simulink model "VehCtrlMdel241025_2018b_amkspdlimit"  (R2019b)
settings: Solver=FixedStepDiscrete  StartTime=0.0  StopTime=30  FixedStep=0.0005  RelTol=1e-3  EnableMultiTasking=on
values from neighbouring files (symbols this model uses):
  Ldwf = 0.4    [VxSpdEstiPara.m]
  Ldwr = 0.5    [VxSpdEstiPara.m]
  thr1 = 0.5    [VxSpdEstiPara.m]
  thr2 = 0.5    [VxSpdEstiPara.m]
  thr3 = 0.5    [VxSpdEstiPara.m]
  thr4 = 0.5    [VxSpdEstiPara.m]
  TrqRquRate = 20    [VxSpdEstiPara.m]
undefined symbols (not defined in the file or in its folder): Ax_OffSet, Ay_OffSet, Caf, Car, DiscIntNeverNeededParam, dwf, dwr, h, i1, i2, I_AN06_5V, I_AN07_5V, I_AN08_5V, I_AN09_5V, I_AN10_5V, I_SW01_L, I_SW02_L, I_SW03_L, I_SW05_L, I_SW07_L, Iz, Kc, Ki, Kp, lf, lr, m, O_SW01_LS0A4, O_SW02_LS0A4, O_SW04_LS0A4, O_SW05_LS0A4, O_SW06_LS0A4, O_SW07_LS0A4, O_SW08_LS0A4, O_SW09_LS0A4, O_SW12_HS1A, O_SW13_HS1A, O_SW14_HS1A, O_SW15_HS1A, Offset_Angle, PWM3, Qa, Ra, RearRatio, Rt, thr5, YawRate_OffSet
libraries: simulink x159, ec5744lib x142, canmsglib x18, MyDesignedModel x1
(part 2 of 6)

== system VehCtrlMdel241025_2018b_amkspdlimit/Input/key ==
  note: 1:cutoff
  function : TriggerPort  TriggerType=function-call  VariantControl=(inherit)
  Acc4 : ec5744lib/RapidECU_U3/01BasicInput/AnalogInput  channel=56:I_AN10_5V  sampletime=-1
      settings: SourceProductName=ECUCoder for MPC5744
  Bus Creator : BusCreator  Inputs=6
  Compare To Constant : simulink/Logic and Bit Operations/Compare To Constant  relop=<=  const=1500  OutDataTypeStr=boolean
  Constant1 : Constant  Value=single(0.11)
  Constant2 : Constant  Commented=on  Value=boolean(1)
  Constant3 : Constant  Value=single(0.11)
  Constant5 : Constant  Value=single(0.11)
  Logical Operator : Logic  Operator=NOT  AllPortsSameDT=off  OutDataTypeStr=boolean
  MeaModule : ec5744lib/RapidECU_U3/07Calibration/MeaModule  signal=TSAL_SW_IN
      settings: SourceProductName=ECUCoder for MPC5744
  MeaModule1 : ec5744lib/RapidECU_U3/07Calibration/MeaModule  signal=ignition
      settings: SourceProductName=ECUCoder for MPC5744
  MeaModule2 : ec5744lib/RapidECU_U3/07Calibration/MeaModule  signal=AMKSWITCH
      settings: SourceProductName=ECUCoder for MPC5744
  MeaModule3 : ec5744lib/RapidECU_U3/07Calibration/MeaModule  signal=HV_voltValid
      settings: SourceProductName=ECUCoder for MPC5744
  SwitchInput : ec5744lib/RapidECU_U3/01BasicInput/SwitchInput  channel=7:I_SW02_L  sampletime=-1
      settings: SourceProductName=ECUCoder for MPC5744
  SwitchInput1 : ec5744lib/RapidECU_U3/01BasicInput/SwitchInput  channel=8:I_SW03_L  sampletime=-1
      settings: SourceProductName=ECUCoder for MPC5744
  SwitchInput2 : ec5744lib/RapidECU_U3/01BasicInput/SwitchInput  channel=10:I_SW05_L  sampletime=-1
      settings: SourceProductName=ECUCoder for MPC5744
  SwitchInput3 : ec5744lib/RapidECU_U3/01BasicInput/SwitchInput  channel=6:I_SW01_L  sampletime=-1
      settings: SourceProductName=ECUCoder for MPC5744
  SwitchInput4 : ec5744lib/RapidECU_U3/01BasicInput/SwitchInput  channel=26:I_SW07_L  sampletime=-1
      settings: SourceProductName=ECUCoder for MPC5744
  Timer : Stateflow chart  TreatAsAtomicUnit=on
  Timer1 : Stateflow chart  TreatAsAtomicUnit=on
  Timer2 : Stateflow chart  TreatAsAtomicUnit=on
  key : Outport  VectorParamsAs1DForOutWhenUnconnected=off
  wires:
  SwitchInput/1 -> Logical Operator/1  "Drive_ready"
  Bus Creator/1 -> key/1
  Logical Operator/1 -> Timer/1(Trigger)  "ignition"
  Constant5/1 -> Timer/2(CountTime)
  Timer/1(Exit) -> MeaModule1/1  "ignition"
  MeaModule1/1 -> Bus Creator/1
  Constant1/1 -> Timer1/2(CountTime)
  Timer1/1(Exit) -> MeaModule2/1  "AMKSWITCH"
  MeaModule2/1 -> Bus Creator/2
  SwitchInput3/1 -> Bus Creator/3  "out2"
  SwitchInput1/1 -> Timer1/1(Trigger)
  Acc4/1 -> Compare To Constant/1  "HV_volt"
  MeaModule/1 -> Bus Creator/4  "TSAL_SW_IN"
  MeaModule3/1 -> Bus Creator/5  "HV_voltValid"
  Compare To Constant/1 -> MeaModule3/1
  SwitchInput4/1 -> Timer2/1(Trigger)
  Timer2/1(Exit) -> Bus Creator/6  "ModeSW"
  Constant3/1 -> Timer2/2(CountTime)
  SwitchInput2/1 -> MeaModule/1  "ignition"

== system VehCtrlMdel241025_2018b_amkspdlimit/Input_Processing/Function-Call Subsystem ==
  INPUT_BUS : Inport
  function : TriggerPort  TriggerType=function-call  VariantControl=Variant
  AccBrkPedal : Subsystem
  Bus Selector : BusSelector  OutputSignals=IMU,AccBrk_BUS,SWAS,ABS_BUS,AMKMCUtoVCU_BUS,AMKMCUtoVCU_BUS.FLAMKMCUtoVCU1,AMKMCUtoVCU_BUS.FRAMKMCUtoVCU1,EMRAXMCU_Receive.MCU_pwr
  Bus Creator : BusCreator  Inputs=6
  IMU : Subsystem
  SWAS : Subsystem
  Subsystem : Subsystem
  Subsystem1 : Subsystem
  Terminator : Terminator
  Terminator1 : Terminator
  Terminator2 : Terminator
  WhlSpdii_mps : Subsystem
  Out1 : Outport  VectorParamsAs1DForOutWhenUnconnected=off
  wires:
  INPUT_BUS/1 -> [BUS], Bus Selector/1  "BUS"
  Bus Selector/1 -> IMU/1(IMU)  "<IMU>"
  Bus Selector/2 -> AccBrkPedal/1(AccBrk_BUS)  "<AccBrk_BUS>"
  Bus Selector/3 -> SWAS/1(SWAS)  "<SWAS>"
  Bus Selector/4 -> WhlSpdii_mps/1(IMU)  "<ABS_BUS>"
  Bus Selector/5 -> Subsystem1/1(In1), WhlSpdii_mps/2(In2)  "<AMKMCUtoVCU_BUS>"
  IMU/1(IMU_BUS) -> Bus Creator/1  "IMU_Processing"
  AccBrkPedal/1(AccBrk) -> Bus Creator/2  "AccBrkPedal_Processing"
  SWAS/1(StrWhlAng&V) -> Bus Creator/3  "SWAS_Processing"
  WhlSpdii_mps/1(WhlSpdii_mps) -> Bus Creator/4  "WhlSpdii_mps"
  Bus Creator/1 -> Out1/1
  [BUS] -> Bus Creator/5
  Bus Selector/6 -> Subsystem/1(In1)  "<FLAMKMCUtoVCU1>"
  Bus Selector/7 -> Subsystem/2(In2)  "<FRAMKMCUtoVCU1>"
  Subsystem/1(Out1) -> Terminator/1
  Subsystem/2(Out2) -> Terminator1/1
  Bus Selector/8 -> Subsystem/3(In3)  "<MCU_pwr>"
  Subsystem/3(Out3) -> Terminator2/1
  Subsystem1/1(AMKerrorTrq_CUT) -> Bus Creator/6  "AMKerrorTrq_CUT"

== system VehCtrlMdel241025_2018b_amkspdlimit/Input_Processing/Subsystem ==
  note: 和实车相反
  note: 信号的滤波去噪应该在其他模块完成
  OutPutBus : Inport
  function : TriggerPort  TriggerType=function-call  VariantControl=(inherit)
  Bus Selector : BusSelector  OutputSignals=WhlSpdii_mps.WhlSpdFL,WhlSpdii_mps.WhlSpdFR,WhlSpdii_mps.WhlSpdRL_mps,WhlSpdii_mps.WhlSpdRR_mps,IMU_Processing.IMU_Yaw_Value,SWAS_Processing.FLWhlStrAng,SWAS_Processing.FRWhlStrAng,IMU_Processing.IMU_Ax_Valid,BUS.IMU.IMU_Ax_Valid,AccBrkPedal_Processing.Acc_POS
  Cast To Double{,1..7} (8 alike) : DataTypeConversion  OutDataTypeStr=single
  From : From  Commented=on  GotoTag=IMU_Aa_mpss
  Gain5 : Gain  Gain=10
  "IntglJudgment " : Subsystem
  MeaModule : ec5744lib/RapidECU_U3/07Calibration/MeaModule  signal=VehVxEst_mps
      settings: SourceProductName=ECUCoder for MPC5744
  Unit Delay : UnitDelay  SampleTime=-1  HasFrameUpgradeWarning=on
  Unit Delay1 : UnitDelay  SampleTime=-1  HasFrameUpgradeWarning=on
  WhlSlpageJudgment : Subsystem
  WhlSpdSelect : Subsystem
  坐标系转换 : Subsystem
  VehVxEst_mps : Outport
  Vxii_mps : Outport  Port=2
  wires:
  Bus Selector/10 -> "IntglJudgment "/8(Acc_POS)  "<Acc_POS>"
  WhlSlpageJudgment/1(WhlSlipFLValid_flag) -> "IntglJudgment "/1(WhlSlipFL_flag), WhlSpdSelect/1(WhlSlipFL_flag)
  WhlSlpageJudgment/5(WhlSpdMax_mps) -> [WhlSpdMax_mps]
  "IntglJudgment "/2(IMUVehSpdEstiExit) -> WhlSpdSelect/8(IMUVehSpdEstiExit)
  WhlSlpageJudgment/2(WhlSlipFRValid_flag) -> "IntglJudgment "/2(WhlSlipFR_flag), WhlSpdSelect/2(WhlSlipFR_flag)
  Bus Selector/8 -> Gain5/1  "<IMU_Ax_Valid>"
  "IntglJudgment "/1(VxIMU_est) -> WhlSpdSelect/7(VxIMU_est)
  WhlSlpageJudgment/3(WhlSlipRLValid_flag) -> "IntglJudgment "/3(WhlSlipRL_flag), WhlSpdSelect/3(WhlSlipRL_flag)
  Cast To Double1/1 -> 坐标系转换/1(WhlSpdFL_mps)
  [IMU_Aa_mpss] -> WhlSpdSelect/6(IMU_Ax_mpss)
  Unit Delay1/1 -> "IntglJudgment "/7(FFVehVxEst_mps)
  [Vxii_mps] -> Vxii_mps/1, WhlSpdSelect/5(Vxii_mps)
  Cast To Double7/1 -> 坐标系转换/7(WhlStrAngR_deg)  "WhlStrAngR_deg"
  Bus Selector/4 -> Cast To Double4/1  "<WhlSpdRR_mps>"
  Cast To Double4/1 -> 坐标系转换/4(WhlSpdRR_mps)
  Cast To Double/1 -> [IMU_Aa_mpss], WhlSlpageJudgment/3(IMU_Aa_mpss)
  Cast To Double2/1 -> 坐标系转换/2(WhlSpdFR_mps)
  [VehVxEst_mps] -> Unit Delay/1
  WhlSlpageJudgment/4(WhlSlipRRValid_flag) -> WhlSpdSelect/4(WhlSlipRR_flag), "IntglJudgment "/4(WhlSlipRR_flag)
  WhlSpdSelect/1(VehVxEst1_mps) -> [VehVxEst_mps], MeaModule/1  "VehVxEst_mps"
  坐标系转换/1(Vxii_mps) -> [Vxii_mps], WhlSlpageJudgment/1(Vxii_mps)  "Vxii_mps"
  Cast To Double5/1 -> 坐标系转换/5(IMU_YawRate_dps)  "IMU_YawRate_dps"
  Cast To Double3/1 -> 坐标系转换/3(WhlSpdRL_mps)
  [VehVxEst_mps] -> Unit Delay1/1
  坐标系转换/2(IMU_YawRate_dps1) -> WhlSlpageJudgment/2(IMU_YawRate_dps)  "IMU_YawRate_dps"
  Bus Selector/3 -> Cast To Double3/1  "<WhlSpdRL_mps>"
  [WhlSpdMax_mps] -> "IntglJudgment "/9(WhlSpdMax_mps)
  Bus Selector/1 -> Cast To Double1/1  "<WhlSpdFL>"
  Bus Selector/2 -> Cast To Double2/1  "<WhlSpdFR>"
  Unit Delay/1 -> WhlSlpageJudgment/4(VehSpdEstiZ1_mps)
  Cast To Double6/1 -> 坐标系转换/6(WhlStrAngL_deg)  "WhlStrAngL_deg"
  Gain5/1 -> Cast To Double/1  "IMU_Ax_mpss"
  Bus Selector/5 -> Cast To Double5/1  "<IMU_Yaw_Value>"
  Bus Selector/6 -> Cast To Double6/1  "<FLWhlStrAng>"
  Bus Selector/7 -> Cast To Double7/1  "<FRWhlStrAng>"
  WhlSpdSelect/2(AccEst_mpss) -> [AccEst_mpss]
  [AccEst_mpss] -> "IntglJudgment "/6(IMU_Ax_mpss)
  OutPutBus/1 -> [OUTPUTBUS], Bus Selector/1
  Bus Selector/9 -> "IntglJudgment "/5(Ax_Valid)  "<IMU_Ax_Valid>"
  [OUTPUTBUS] -> WhlSlpageJudgment/5(In5)
  MeaModule/1 -> VehVxEst_mps/1

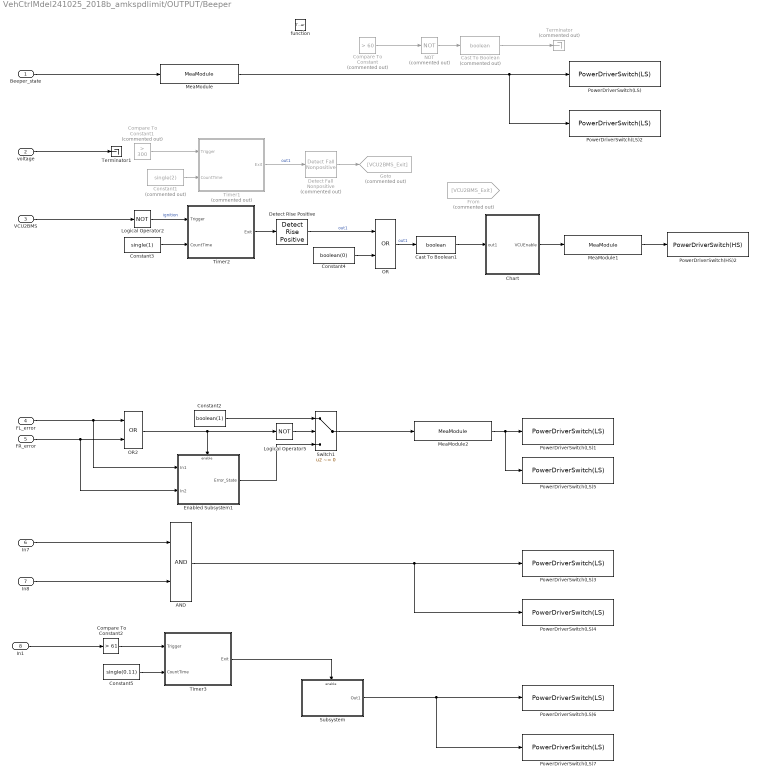
== system VehCtrlMdel241025_2018b_amkspdlimit/OUTPUT/Beeper ==
  Beeper_state : Inport
  voltage : Inport  Port=2
  VCU2BMS : Inport  Port=3
  FL_error : Inport  Port=4
  FR_error : Inport  Port=5
  In7 : Inport  Port=6
  In8 : Inport  Port=7
  In1 : Inport  Port=8
  function : TriggerPort  TriggerType=function-call  VariantControl=(inherit)
  AND : Logic  AllPortsSameDT=off  OutDataTypeStr=boolean
  Cast To Boolean : DataTypeConversion  Commented=on  OutDataTypeStr=boolean
  Cast To Boolean1 : DataTypeConversion  OutDataTypeStr=boolean
  Chart : Stateflow chart  BlockKeywords=__PRM__SERIALIZED__DATA__:Stateflow Chart,Stateflow Diagram  TreatAsAtomicUnit=on
  Compare To Constant : simulink/Logic and Bit Operations/Compare To Constant  Commented=on  relop=>  const=60  OutDataTypeStr=boolean
  Compare To Constant1 : simulink/Logic and Bit Operations/Compare To Constant  Commented=on  relop=>  const=300  OutDataTypeStr=boolean
  Compare To Constant2 : simulink/Logic and Bit Operations/Compare To Constant  relop=>  const=61  OutDataTypeStr=boolean
  Constant1 : Constant  Commented=on  Value=single(2)
  Constant2 : Constant  Value=boolean(1)
  Constant3 : Constant  Value=single(1)
  Constant4 : Constant  Value=boolean(0)
  Constant5 : Constant  Value=single(0.11)
  Detect Fall Nonpositive : simulink/Logic and Bit Operations/Detect Fall Nonpositive  Commented=on  vinit=1  OutDataTypeStr=boolean
      settings: SourceProductName=Simulink  SourceProductBaseCode=SL
  Detect Rise Positive : simulink/Logic and Bit Operations/Detect Rise Positive  vinit=0  OutDataTypeStr=boolean
  Enabled Subsystem1 : Subsystem  TreatAsAtomicUnit=on
  From : From  Commented=on  GotoTag=VCU2BMS_Exit
  Goto : Goto  Commented=on  GotoTag=VCU2BMS_Exit
  Logical Operator2 : Logic  Operator=NOT  AllPortsSameDT=off  OutDataTypeStr=boolean
  Logical Operator5 : Logic  Operator=NOT  AllPortsSameDT=off  OutDataTypeStr=boolean
  MeaModule : ec5744lib/RapidECU_U3/07Calibration/MeaModule  signal=beeper_state
      settings: SourceProductName=ECUCoder for MPC5744
  MeaModule1 : ec5744lib/RapidECU_U3/07Calibration/MeaModule  signal=HVSWITCH
      settings: SourceProductName=ECUCoder for MPC5744
  MeaModule2 : ec5744lib/RapidECU_U3/07Calibration/MeaModule  signal=STATEDISPLAY
      settings: SourceProductName=ECUCoder for MPC5744
  NOT : Logic  Commented=on  Operator=NOT  AllPortsSameDT=off  OutDataTypeStr=boolean
  OR : Logic  Operator=OR  AllPortsSameDT=off  OutDataTypeStr=boolean
  OR2 : Logic  Operator=OR  AllPortsSameDT=off  OutDataTypeStr=boolean
  PowerDriverSwitch(HS)2 : ec5744lib/RapidECU_U3/02PowerDriverSwitch/PowerDriverSwitch(HS)  channel=115:O_SW13_HS1A  sampletime=-1
      settings: SourceProductName=ECUCoder for MPC5744
  PowerDriverSwitch(LS) : ec5744lib/RapidECU_U3/02PowerDriverSwitch/PowerDriverSwitch(LS)  channel=78:O_SW05_LS0A4  sampletime=-1
      settings: SourceProductName=ECUCoder for MPC5744
  PowerDriverSwitch(LS)1 : ec5744lib/RapidECU_U3/02PowerDriverSwitch/PowerDriverSwitch(LS)  channel=63:O_SW04_LS0A4  sampletime=-1
      settings: SourceProductName=ECUCoder for MPC5744
  PowerDriverSwitch(LS)2 : ec5744lib/RapidECU_U3/02PowerDriverSwitch/PowerDriverSwitch(LS)  channel=79:O_SW06_LS0A4  sampletime=-1
      settings: SourceProductName=ECUCoder for MPC5744
  PowerDriverSwitch(LS)3 : ec5744lib/RapidECU_U3/02PowerDriverSwitch/PowerDriverSwitch(LS)  channel=82:O_SW07_LS0A4  sampletime=-1
      settings: SourceProductName=ECUCoder for MPC5744
  PowerDriverSwitch(LS)4 : ec5744lib/RapidECU_U3/02PowerDriverSwitch/PowerDriverSwitch(LS)  channel=91:O_SW08_LS0A4  sampletime=-1
      settings: SourceProductName=ECUCoder for MPC5744
  PowerDriverSwitch(LS)5 : ec5744lib/RapidECU_U3/02PowerDriverSwitch/PowerDriverSwitch(LS)  channel=92:O_SW09_LS0A4  sampletime=-1
      settings: SourceProductName=ECUCoder for MPC5744
  PowerDriverSwitch(LS)6 : ec5744lib/RapidECU_U3/02PowerDriverSwitch/PowerDriverSwitch(LS)  channel=58:O_SW01_LS0A4  sampletime=-1
      settings: SourceProductName=ECUCoder for MPC5744
  PowerDriverSwitch(LS)7 : ec5744lib/RapidECU_U3/02PowerDriverSwitch/PowerDriverSwitch(LS)  channel=59:O_SW02_LS0A4  sampletime=-1
      settings: SourceProductName=ECUCoder for MPC5744
  Subsystem : Subsystem
  Switch1 : Switch  Criteria=u2 ~= 0
  Terminator : Terminator  Commented=on
  Terminator1 : Terminator
  Timer1 : Stateflow chart  Commented=on  TreatAsAtomicUnit=on
  Timer2 : Stateflow chart  TreatAsAtomicUnit=on
  Timer3 : Stateflow chart  TreatAsAtomicUnit=on
  wires:
  Beeper_state/1 -> MeaModule/1
  MeaModule/1 -> PowerDriverSwitch(LS)2/1, PowerDriverSwitch(LS)/1
  voltage/1 -> Terminator1/1
  Compare To Constant/1 -> NOT/1
  NOT/1 -> Cast To Boolean/1
  Cast To Boolean/1 -> Terminator/1
  Constant1/1 -> Timer1/2(CountTime)
  Compare To Constant1/1 -> Timer1/1(Trigger)
  Detect Fall Nonpositive/1 -> Goto/1
  OR/1 -> Cast To Boolean1/1  "out1"
  Timer2/1(Exit) -> Detect Rise Positive/1
  Logical Operator2/1 -> Timer2/1(Trigger)  "ignition"
  Chart/1(VCUEnable) -> MeaModule1/1
  Cast To Boolean1/1 -> Chart/1(out1)
  Constant3/1 -> Timer2/2(CountTime)
  VCU2BMS/1 -> Logical Operator2/1
  Detect Rise Positive/1 -> OR/1  "out1"
  Constant4/1 -> OR/2
  Timer1/1(Exit) -> Detect Fall Nonpositive/1  "out1"
  OR2/1 -> Logical Operator5/1, Enabled Subsystem1/Enable
  Constant2/1 -> Switch1/1
  Logical Operator5/1 -> Switch1/2
  FL_error/1 -> Enabled Subsystem1/1(In1), OR2/1
  Enabled Subsystem1/1(Error_State) -> Switch1/3
  Switch1/1 -> MeaModule2/1
  FR_error/1 -> Enabled Subsystem1/2(In2), OR2/2
  MeaModule1/1 -> PowerDriverSwitch(HS)2/1
  MeaModule2/1 -> PowerDriverSwitch(LS)5/1, PowerDriverSwitch(LS)1/1
  In8/1 -> AND/2
  In7/1 -> AND/1
  AND/1 -> PowerDriverSwitch(LS)4/1, PowerDriverSwitch(LS)3/1
  Compare To Constant2/1 -> Timer3/1(Trigger)
  Constant5/1 -> Timer3/2(CountTime)
  In1/1 -> Compare To Constant2/1
  Timer3/1(Exit) -> Subsystem/Enable
  Subsystem/1(Out1) -> PowerDriverSwitch(LS)7/1, PowerDriverSwitch(LS)6/1

== system VehCtrlMdel241025_2018b_amkspdlimit/OUTPUT/VCU2AMKMCUFL ==
  MCFL_TargetTorque : Inport
  In2 : Inport  Port=2
  function : TriggerPort  TriggerType=function-call  VariantControl=(inherit)
  Bus Selector : BusSelector  OutputSignals=MCFL_TorqueOn,MCFL_DCOn_setpoints,MCFL_DCEnable,errorReset,MCFL_InverterOn
  CAN Pack1 : canmsglib/CAN Pack  CANdbFile=d:\Users\YJR\Desktop\低压组\amk电机\DRe20_dbc_v1.16\DRe20_dbc_v1.16_CAN2.dbc  MsgList=(none)  MsgName=MCFL_SetPoints  MsgIDType=Standard (11-bit identifier)  MsgIdentifier=386  MsgLength=8  Remote=off  ApplyMinMax=off  BusOutput=off  SignalInfo={'MCFL_TargetTorque','16','16','LE','signed','Standard','0','0.0098','0','-Inf','Inf';'MCFL_TorqueLimitN','48','16','LE','signed','Standard','0','0.0098','0','-Inf','Inf';'MCFL_TorqueLimitP','32','16','LE','signed','Standard','0','0.0098','0','-Inf','Inf';'MCFL_cDCOn','9','1','LE','unsigned','Standard','0','1','0','0','1';'MCFL_cEnable','10','1','LE','unsigned','Standard','0','1','0','0','1';'MCFL_cErrorReset','11','1','LE','unsigned','Standard','0','1','0','0','1';'MCFL_cInverterOn','8','1','LE','unsigned','Standard','0','1','0','0','1';'MCFL_cReserve1','0','8','LE','unsigned','Standard','0','1','0','-Inf','Inf';'MCFL_cReserve2','12','4','LE','unsigned','Standard','0','1','0','-Inf','Inf'}
      settings: SourceProductName=Vehicle Network Toolbox  SourceProductBaseCode=VN  DataFormat=CANdb specified signals
  CANPackMessage : ec5744lib/RapidECU_U3/04CANCommunication/CANPackMessage  datalength=8  sampletime=-1
      settings: SourceProductName=ECUCoder for MPC5744
  CANTransmit : ec5744lib/RapidECU_U3/04CANCommunication/CANTransmit  canmodule=1  canbuffer=8  canmessageid=386  canmessagetype=Standard(11-bit ID)  datalength=8  sampletime=-1
      settings: SourceProductName=ECUCoder for MPC5744
  Constant1 : Constant  Value=0
  Constant2 : Constant  Value=21
  Gain : Gain  Gain=-1
  Ground1 : Ground
  Ground2 : Ground
  Switch : Switch  Criteria=u2 ~= 0
  Switch1 : Switch  Criteria=u2 ~= 0
  Terminator3 : Terminator
  wires:
  CANPackMessage/1 -> CANTransmit/1
  CAN Pack1/1 -> CANPackMessage/1
  CANTransmit/1 -> Terminator3/1
  MCFL_TargetTorque/1 -> CAN Pack1/1  "MCFL_TargetTorque"
  Constant1/1 -> Switch/3, Switch1/3
  Bus Selector/2 -> CAN Pack1/4  "<MCFL_DCOn_setpoints>"
  Switch/1 -> CAN Pack1/3  "MCFL_TorqueLimitP"
  Ground1/1 -> CAN Pack1/8  "MCFL_cReserve1"
  Bus Selector/5 -> CAN Pack1/7  "<MCFL_InverterOn>"
  Bus Selector/3 -> CAN Pack1/5  "<MCFL_DCEnable>"
  Ground2/1 -> CAN Pack1/9  "MCFL_cReserve2"
  In2/1 -> Bus Selector/1
  Bus Selector/4 -> CAN Pack1/6  "<errorReset>"
  Bus Selector/1 -> Switch1/2, Switch/2  "<MCFL_TorqueOn>"
  Constant2/1 -> Switch/1, Gain/1
  Gain/1 -> Switch1/1
  Switch1/1 -> CAN Pack1/2

== system VehCtrlMdel241025_2018b_amkspdlimit/OUTPUT/VCU2AMKMCUFR ==
  <BUS> : Inport
  In1 : Inport  Port=2
  function : TriggerPort  TriggerType=function-call  VariantControl=(inherit)
  Bus Selector : BusSelector  OutputSignals=MCFR_TorqueOn,MCFL_DCOn_setpoints,MCFL_DCEnable,errorReset,MCFL_InverterOn
  CAN Pack1 : canmsglib/CAN Pack  CANdbFile=C:\Users\12045\Desktop\DBC\DRe20_dbc_v1.16\DRe20_dbc_v1.16_CAN2.dbc  MsgList=MCFR_SetPoints  MsgName=MCFR_SetPoints  MsgIDType=Standard (11-bit identifier)  MsgIdentifier=387  MsgLength=8  Remote=off  ApplyMinMax=off  BusOutput=off  SignalInfo={'MCFR_TargetTorque','16','16','LE','signed','Standard','0','0.0098','0','-Inf','Inf';'MCFR_TorqueLimitN','48','16','LE','signed','Standard','0','0.0098','0','-Inf','Inf';'MCFR_TorqueLimitP','32','16','LE','signed','Standard','0','0.0098','0','-Inf','Inf';'MCFR_cDCOn','9','1','LE','unsigned','Standard','0','1','0','0','1';'MCFR_cEnable','10','1','LE','unsigned','Standard','0','1','0','0','1';'MCFR_cErrorReset','11','1','LE','unsigned','Standard','0','1','0','0','1';'MCFR_cInverterOn','8','1','LE','unsigned','Standard','0','1','0','0','1';'MCFR_cReserve1','0','8','LE','unsigned','Standard','0','1','0','-Inf','Inf';'MCFR_cReserve2','12','4','LE','unsigned','Standard','0','1','0','-Inf','Inf'}
      settings: SourceProductName=Vehicle Network Toolbox  SourceProductBaseCode=VN  DataFormat=CANdb specified signals
  CANPackMessage : ec5744lib/RapidECU_U3/04CANCommunication/CANPackMessage  datalength=8  sampletime=-1
      settings: SourceProductName=ECUCoder for MPC5744
  CANTransmit : ec5744lib/RapidECU_U3/04CANCommunication/CANTransmit  canmodule=1  canbuffer=9  canmessageid=387  canmessagetype=Standard(11-bit ID)  datalength=8  sampletime=-1
      settings: SourceProductName=ECUCoder for MPC5744
  Constant : Constant  Value=0
  Constant1 : Constant  Value=21
  Gain : Gain  Gain=-1
  Ground : Ground
  Ground1 : Ground
  Switch : Switch  Criteria=u2 ~= 0
  Switch1 : Switch  Criteria=u2 ~= 0
  Terminator3 : Terminator
  wires:
  Ground1/1 -> CAN Pack1/9  "MCFR_cReserve2"
  Bus Selector/3 -> CAN Pack1/5  "<MCFL_DCEnable>"
  Bus Selector/4 -> CAN Pack1/6  "<errorReset>"
  Bus Selector/5 -> CAN Pack1/7  "<MCFL_InverterOn>"
  Ground/1 -> CAN Pack1/8  "MCFR_cReserve1"
  Switch/1 -> CAN Pack1/3
  Bus Selector/2 -> CAN Pack1/4  "<MCFL_DCOn_setpoints>"
  Constant/1 -> Switch/3, Switch1/3
  CANTransmit/1 -> Terminator3/1
  CAN Pack1/1 -> CANPackMessage/1
  CANPackMessage/1 -> CANTransmit/1
  In1/1 -> CAN Pack1/1
  <BUS>/1 -> Bus Selector/1
  Constant1/1 -> Switch/1, Gain/1
  Bus Selector/1 -> Switch/2, Switch1/2  "<MCFR_TorqueOn>"
  Switch1/1 -> CAN Pack1/2
  Gain/1 -> Switch1/1

== system VehCtrlMdel241025_2018b_amkspdlimit/OUTPUT/VCU2CLUSTER ==
  In1 : Inport
  TCS : Inport  Port=2
  function : TriggerPort  TriggerType=function-call  VariantControl=Variant
  Bus Selector : BusSelector  OutputSignals=signal2.APPBrk_BUS.Brk_F,signal2.MCU.MCU_state.Trq,signal2.APPBrk_BUS.Acc_POS,signal2.MCU.MCU_pwr.motor_temp,signal2.VehSpd_FLkph,signal2.MCU.MCU_state.Spd_R_kph,signal2.APPBrk_BUS.Brk_R,signal2.MCU.MCU_state.RPM
  Bus Selector1 : BusSelector  OutputSignals=TCS_TrqRequestFinal_Nm,TCS_flgActv
  CAN Pack : canmsglib/CAN Pack  CANdbFile=E:\candbc\cluster.dbc  MsgList=(none)  MsgName=New_Message_1  MsgIDType=Standard (11-bit identifier)  MsgIdentifier=291  MsgLength=8  Remote=off  ApplyMinMax=off  BusOutput=off  SignalInfo={'Brk_F','56','8','LE','signed','Standard','0','30','100','-3740','3910';'TCS_Trq_cmd','40','8','LE','unsigned','Standard','0','1','0','0','255';'TCS_flag','32','8','LE','signed','Standard','0','1','0','-Inf','Inf';'Trq_feedback','48','8','LE','signed','Standard','0','1','0','-128','250';'acc','24','8','LE','unsigned','Standard','0','1','0','0','100';'motor_temp','0','8','LE','unsigned','Standard','0','1','0','0','100';'veh_spd_F','8','8','LE','unsigned','Standard','0','1','0','0','120';'veh_spd_R','16','8','LE','unsigned','Standard','0','1','0','0','120'}
      settings: SourceProductName=Vehicle Network Toolbox  SourceProductBaseCode=VN  DataFormat=CANdb specified signals
  CAN Pack1 : canmsglib/CAN Pack  CANdbFile=E:\candbc\cluster.dbc  MsgList=(none)  MsgName=New_Message_2  MsgIDType=Standard (11-bit identifier)  MsgIdentifier=292  MsgLength=2  Remote=off  ApplyMinMax=off  BusOutput=off  SignalInfo={'Brk_R','0','8','LE','signed','Standard','0','30','100','-Inf','Inf';'RPM_feedback','8','8','LE','signed','Standard','0','1','0','-Inf','Inf'}
      settings: SourceProductName=Simulink Real-Time  SourceProductBaseCode=XP  DataFormat=CANdb specified signals
  CANPackMessage : ec5744lib/RapidECU_U3/04CANCommunication/CANPackMessage  datalength=8  sampletime=-1
      settings: SourceProductName=ECUCoder for MPC5744
  CANPackMessage1 : ec5744lib/HYFCU001/04CANCommunication/CANPackMessage  datalength=8  sampletime=-1
      settings: SourceProductName=ECUCoder for MPC5744
  CANTransmit : ec5744lib/RapidECU_U3/04CANCommunication/CANTransmit  canmodule=0  canbuffer=9  canmessageid=291  canmessagetype=Standard(11-bit ID)  datalength=8  sampletime=-1
      settings: SourceProductName=ECUCoder for MPC5744
  CANTransmit1 : ec5744lib/RapidECU_U3/04CANCommunication/CANTransmit  canmodule=0  canbuffer=10  canmessageid=292  canmessagetype=Standard(11-bit ID)  datalength=8  sampletime=-1
      settings: SourceProductName=ECUCoder for MPC5744
  Terminator1 : Terminator
  Terminator3 : Terminator
  wires:
  CANTransmit/1 -> Terminator3/1
  CANPackMessage/1 -> CANTransmit/1
  CAN Pack/1 -> CANPackMessage/1
  In1/1 -> Bus Selector/1
  Bus Selector/5 -> CAN Pack/7  "<VehSpd_FLkph>"
  Bus Selector/4 -> CAN Pack/6  "<motor_temp>"
  Bus Selector/3 -> CAN Pack/5  "<Acc_POS>"
  Bus Selector/6 -> CAN Pack/8  "<Spd_R_kph>"
  Bus Selector/1 -> CAN Pack/1  "<Brk_F>"
  Bus Selector/2 -> CAN Pack/4  "<Trq>"
  TCS/1 -> Bus Selector1/1
  Bus Selector1/2 -> CAN Pack/3  "<TCS_flgActv>"
  Bus Selector1/1 -> CAN Pack/2  "<TCS_TrqRequestFinal_Nm>"
  Bus Selector/7 -> CAN Pack1/1  "<Brk_R>"
  Bus Selector/8 -> CAN Pack1/2  "<RPM>"
  CAN Pack1/1 -> CANPackMessage1/1
  CANPackMessage1/1 -> CANTransmit1/1
  CANTransmit1/1 -> Terminator1/1

== system VehCtrlMdel241025_2018b_amkspdlimit/OUTPUT/VCU2EmraxMCU ==
  note: 0: 0Nm
      | 2: Trq mode
  note: 0: N
      | 2:D
  note: 加ramp
  note: 1.spd改成motor_rpm
      | 2.APP_bad改成acc_error
      | 3.设置模式的优先级
      | 4.车轮低负载（悬空），加最高车速限制
  In1 : Inport
  function : TriggerPort  TriggerType=function-call  VariantControl=(inherit)
  Bus Selector : BusSelector  OutputSignals=Trq_CUT,VCU_SpdCmd_Emrax,TrqR_cmd
  CAN Pack1 : canmsglib/CAN Pack  CANdbFile=E:\candbc\MCU_No1.dbc  MsgList=(none)  MsgName=VCU2MCU1_ID1  MsgIDType=Extended (29-bit identifier)  MsgIdentifier=146927393  MsgLength=8  Remote=off  ApplyMinMax=off  BusOutput=off  SignalInfo={'VCU2MCU_Control_mode_ID1','32','8','LE','unsigned','Standard','0','1','0','0','255';'VCU2MCU_Gear_ID1','40','2','LE','unsigned','Standard','0','1','0','0','3';'VCU2MCU_Speed_Limit_ID1','0','16','LE','unsigned','Standard','0','5.000000e-01','-10000','-10000','10000';'VCU2MCU_Torque_Control_ID1','16','16','LE','unsigned','Standard','0','1','0','0','1000'}
      settings: SourceProductName=Vehicle Network Toolbox  SourceProductBaseCode=VN  DataFormat=CANdb specified signals
  CANPackMessage : ec5744lib/RapidECU_U3/04CANCommunication/CANPackMessage  datalength=8  sampletime=-1
      settings: SourceProductName=ECUCoder for MPC5744
  CANTransmit : ec5744lib/RapidECU_U3/04CANCommunication/CANTransmit  canmodule=0  canbuffer=8  canmessageid=146927393  canmessagetype=Extended(29-bit ID)  datalength=8  sampletime=-1
      settings: SourceProductName=ECUCoder for MPC5744
  Cast To Boolean4 : DataTypeConversion  OutDataTypeStr=single
  Cast To Boolean6 : DataTypeConversion  OutDataTypeStr=single
  Constant13 : Constant  Value=2
  Constant17 : Constant  Value=0
  Constant19 : Constant  Value=2
  Constant20 : Constant  Value=0
  Data Type Conversion1 : DataTypeConversion  OutDataTypeStr=single
  Data Type Conversion2 : DataTypeConversion  OutDataTypeStr=int32
  MeaModule1 : ec5744lib/HYFCU001/07Calibration/MeaModule  signal=Gear_Trs
      settings: SourceProductName=ECUCoder for MPC5744
  MeaModule2 : ec5744lib/HYFCU001/07Calibration/MeaModule  signal=Mode_Trs
      settings: SourceProductName=ECUCoder for MPC5744
  Ramp : simulink/Sources/Ramp  Commented=on  slope=1  start=0  InitialOutput=0
  Switch2 : Switch  Criteria=u2 > Threshold
  Switch3 : Switch  Criteria=u2 > Threshold
  Terminator3 : Terminator
  wires:
  CANTransmit/1 -> Terminator3/1
  CAN Pack1/1 -> CANPackMessage/1
  CANPackMessage/1 -> CANTransmit/1
  MeaModule1/1 -> Cast To Boolean4/1
  Bus Selector/2 -> Data Type Conversion1/1  "<VCU_SpdCmd_Emrax>"
  Constant20/1 -> Switch2/1
  Bus Selector/1 -> Switch2/2, Switch3/2  "<Trq_CUT>"
  Constant19/1 -> Switch2/3
  Constant13/1 -> Switch3/3
  Constant17/1 -> Switch3/1
  Switch3/1 -> MeaModule2/1
  Switch2/1 -> MeaModule1/1
  MeaModule2/1 -> Cast To Boolean6/1
  Data Type Conversion1/1 -> CAN Pack1/3
  Data Type Conversion2/1 -> CAN Pack1/4
  Cast To Boolean4/1 -> CAN Pack1/1
  Cast To Boolean6/1 -> CAN Pack1/2
  Bus Selector/3 -> Data Type Conversion2/1  "<TrqR_cmd>"
  In1/1 -> Bus Selector/1

== system VehCtrlMdel241025_2018b_amkspdlimit/OUTPUT/WP_OUTPUT ==
  note: 数据类型转换
  aWaterPumpON : Inport
  bWaterPumpON : Inport  Port=2
  LoadOfbWaterPump : Inport  Port=3
  function : TriggerPort  TriggerType=function-call  VariantControl=(inherit)
  Cast To Single : DataTypeConversion  OutDataTypeStr=boolean
  Cast To Single1 : DataTypeConversion  OutDataTypeStr=uint16
  Cast To Single2 : DataTypeConversion  OutDataTypeStr=boolean
  Constant : Constant  Value=uint16(1000)  OutDataTypeStr=uint16  SampleTime=-1
  PowerDriverPWM : ec5744lib/RapidECU_U3/03PowerDriverPWM/PowerDriverPWM  channel=114:O_SW12_HS1A/PWM3  sampletime=-1
      settings: SourceProductName=ECUCoder for MPC5744
  PowerDriverSwitch(HS) : ec5744lib/RapidECU_U3/02PowerDriverSwitch/PowerDriverSwitch(HS)  channel=117:O_SW14_HS1A  sampletime=-1
      settings: SourceProductName=ECUCoder for MPC5744
  PowerDriverSwitch(HS)1 : ec5744lib/RapidECU_U3/02PowerDriverSwitch/PowerDriverSwitch(HS)  channel=118:O_SW15_HS1A  sampletime=-1
      settings: SourceProductName=ECUCoder for MPC5744
  wires:
  LoadOfbWaterPump/1 -> Cast To Single1/1
  Constant/1 -> PowerDriverPWM/1
  aWaterPumpON/1 -> Cast To Single/1
  Cast To Single/1 -> PowerDriverSwitch(HS)/1
  Cast To Single1/1 -> PowerDriverPWM/2
  bWaterPumpON/1 -> Cast To Single2/1
  Cast To Single2/1 -> PowerDriverSwitch(HS)1/1

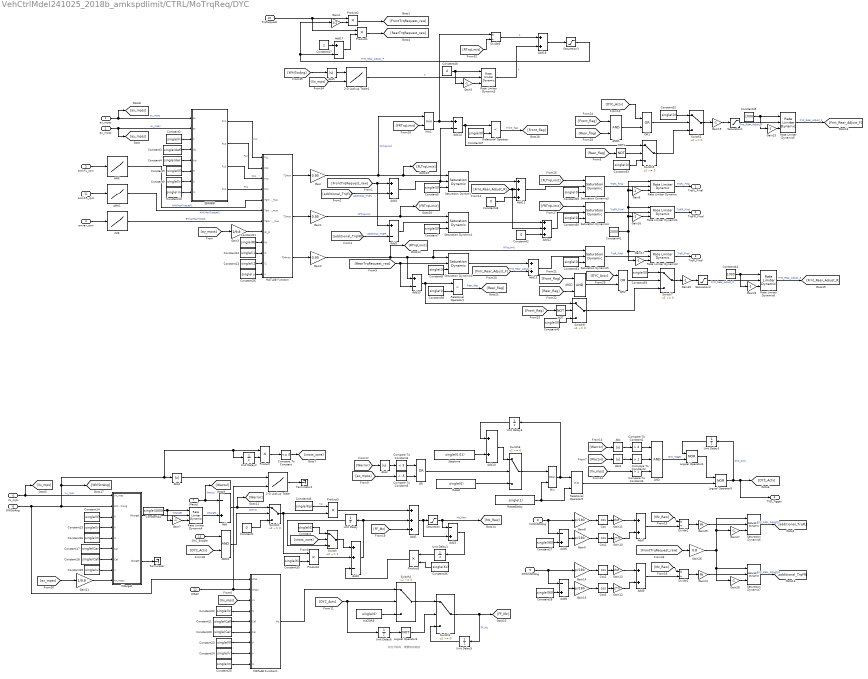
== system VehCtrlMdel241025_2018b_amkspdlimit/CTRL/MoTrqReq/DYC ==
  note: 积分开始时，需要给初始值
  ax_mpss : Inport
  ay_mpss : Inport  Port=2
  amkFL_rpm : Inport  Port=3
  emrax_rpm : Inport  Port=4
  Vx_mps : Inport  Port=5
  WhlStrAng : Inport  Port=6
  Wactul : Inport  Port=7
  FLWhlStrAng : Inport  Port=8
  FRWhlStrAng : Inport  Port=9
  TrqRequest : Inport  Port=10
  amkFR_rpm : Inport  Port=11
  WSAV : Inport  Port=12
  DYC_Enable : Inport  Port=13
  2-D Lookup Table : Lookup_n-D  BreakpointsForDimension1=[0 5 20 25]  BreakpointsForDimension2=[20 40 60]  Table=[3 5 8;5 8 10;6 10 13;8 12 14]  InternalRulePriority=Speed  RndMeth=Simplest  InputSameDT=on
  2-D Lookup Table1 : Lookup_n-D  BreakpointsForDimension1=[0;5;20;25;30]  BreakpointsForDimension2=[0;5;8;10;20;40;60]  Table=[0 0 0 0 0 0 0;0 0.3 0.45 0.5 0.53 0.55 0.58;0 0.4 0.55 0.56 0.58 0.62 0.65;0 0.55 0.7 0.72 0.78 0.81 0.83;0 0.6 0.8 0.82 0.86 0.89 0.9]  InternalRulePriority=Speed  RndMeth=Simplest  InputSameDT=on
  228 : Lookup_n-D  NumberOfTableDimensions=1  BreakpointsForDimension1=[200;400;600;800;1000;1200;1400;1600;1800;2000;2200;2400;2600;2800;3000;3200;3400;3600;3800;4000;4200;4400;4600;4800;5000;5200;5400]  BreakpointsForDimension2=[1:3]  Table=[229.85;229.85;229.85;229.85;229.85;229.85;229.85;229.85;229.85;229.85;229.85;229.85;229.46;229.16;228.86;228.86;228.86;228.86;228.86;227.86;227.86;226.87;225.86;224.86;220.86;218.87;215.87]  InternalRulePriority=Speed  RndMeth=Simplest  InputSameDT=on
  AMK : Lookup_n-D  NumberOfTableDimensions=1  BreakpointsForDimension1=[0;1000;2000;3000;4000;5000;6000;7000;8000;9000;10000;11000;12000;13000;14000;15000;16000;17000;18000;19000]  BreakpointsForDimension2=[1:3]  Table=[21;21;21;21;21;21;21;21;21;21;21;21;21;21;20;17.5;15;12.5;8;0]  InternalRulePriority=Speed  RndMeth=Simplest  InputSameDT=on
  AMK1 : Lookup_n-D  NumberOfTableDimensions=1  BreakpointsForDimension1=[0;1000;2000;3000;4000;5000;6000;7000;8000;9000;10000;11000;12000;13000;14000;15000;16000;17000;18000;19000]  BreakpointsForDimension2=[1:3]  Table=[21;21;21;21;21;21;21;21;21;21;21;21;21;21;20;17.5;15;12.5;8;0]  InternalRulePriority=Speed  RndMeth=Simplest  InputSameDT=on
  AND : Logic  Inputs=3  AllPortsSameDT=off  OutDataTypeStr=boolean
  AND1 : Logic  AllPortsSameDT=off  OutDataTypeStr=boolean
  AND2 : Logic  AllPortsSameDT=off  OutDataTypeStr=boolean
  AND3 : Logic  AllPortsSameDT=off  OutDataTypeStr=boolean
  Abs{,1..2,4..5} (5 alike) : Abs
  Add{,3,6,8} (4 alike) : Sum  Inputs=-+
  Add1 : Sum  Inputs=+++
  Add{4,7,9..10,13,18} (6 alike) : Sum
  Add11 : Sum  Inputs=+++
  Add12 : Sum  Inputs=+++
  Add{5,14..15,17} (4 alike) : Sum  Inputs=+-
  Add2 : Sum  Inputs=++-
  Compare To Constant : simulink/Logic and Bit Operations/Compare To Constant  relop=<=  const=0  OutDataTypeStr=boolean
  Compare To Constant1 : simulink/Logic and Bit Operations/Compare To Constant  relop=>  const=4  OutDataTypeStr=boolean
  Compare To Constant2 : simulink/Logic and Bit Operations/Compare To Constant  relop=>  const=1  OutDataTypeStr=boolean
  Compare To Constant3 : simulink/Logic and Bit Operations/Compare To Constant  relop=>  const=2  OutDataTypeStr=boolean
  Compare To Constant4 : simulink/Logic and Bit Operations/Compare To Constant  relop=<  const=3  OutDataTypeStr=boolean
  Compare To Constant5 : simulink/Logic and Bit Operations/Compare To Constant  relop=<  const=-5  OutDataTypeStr=boolean
  Constant{,6..8,29..33,37..40} (13 alike) : Constant  Value=single(0)
  Constant1 : Constant  Value=0
  Constant10 : Constant  Value=single(m)
  Constant11 : Constant  Value=single(Rt)
  Constant12 : Constant  Value=single(i1)
  Constant13 : Constant  Value=single(i2)
  Constant14 : Constant  Value=single(lf)
  Constant15 : Constant  Value=single(lr)
  Constant16 : Constant  Value=single(m)
  Constant17 : Constant  Value=single(Car)
  Constant18 : Constant  Value=single(Caf)
  Constant19 : Constant  Value=single(u)
  Constant2 : Constant  Value=single(h)
  Constant20 : Constant  Value=single(Car)
  Constant21 : Constant  Value=single(Caf)
  Constant22 : Constant  Value=single(Iz)
  Constant23 : Constant  Value=single(lf)
  Constant24 : Constant  Value=single(lr)
  Constant25 : Constant  Value=single(m)
  Constant26 : Constant  Value=single(u)
  Constant27 : Constant  Value=single(90)
  Constant28 : Constant  Value=single(90)
  Constant3 : Constant  Value=single(dwf)
  Constant34 : Constant  Value=single(4000)
  Constant35 : Constant  Value=single(Ki)
  Constant36 : Constant  Value=single(Kc)
  Constant4 : Constant  Value=single(dwr)
  Constant41 : Constant  Value=2000
  Constant42 : Constant  Value=0
  Constant43 : Constant  Value=0
  Constant44 : Constant  Value=1000
  Constant45 : Constant  Value=1000
  Constant46 : Constant  Value=single(Kp)
  Constant47 : Constant
  Constant48 : Constant  Value=4
  Constant5 : Constant  Value=single(lf)
  Constant9 : Constant  Value=single(lr)
  Cos{,1..3} (4 alike) : Trigonometry  Operator=cos
  Divide1 : Product  Inputs=*/
  Divide2 : Product  Inputs=*/
  Divide3 : Product  Inputs=*/
  Gain : Gain  Gain=0.95
  Gain1 : Gain  Gain=0.95
  Gain10 : Gain  Gain=2*lf
  Gain11 : Gain  Gain=dwf
  Gain12 : Gain  Gain=2*lf
  Gain13 : Gain  Gain=dwf
  Gain{8..9,14..15} (4 alike) : Gain  Gain=pi/180
  Gain{5..7,16..17,19..20,22..23,27..28} (11 alike) : Gain  Gain=-1
  Gain2 : Gain  Gain=0.95
  Gain21 : Gain  Gain=1/9.8
  Gain24 : Gain  Gain=Rt
  Gain25 : Gain  Gain=Rt
  Gain26 : Gain  Gain=0.8
  Gain3 : Gain  Gain=1/9.8
  Gain4 : Gain  Gain=1/2
  InitZORE : Constant  Value=single(0)
  Logical Operator3 : Logic  Operator=NOT  AllPortsSameDT=off  OutDataTypeStr=boolean
  Logical Operator4 : Logic  Operator=NOR  AllPortsSameDT=off  OutDataTypeStr=boolean
  Logical Operator5 : Logic  Operator=NOR  AllPortsSameDT=off  OutDataTypeStr=boolean
  MATLAB Function : MATLAB Function  TreatAsAtomicUnit=on
  MATLAB Function1 : MATLAB Function  TreatAsAtomicUnit=on
  Min : MinMax  Inputs=2
  Min1 : MinMax  Inputs=2
  NOT : Logic  Operator=NOT  AllPortsSameDT=off  OutDataTypeStr=boolean
  NOT1 : Logic  Operator=NOT  AllPortsSameDT=off  OutDataTypeStr=boolean
  OR : Logic  Operator=OR  AllPortsSameDT=off  OutDataTypeStr=boolean
  OR1 : Logic  Operator=OR  AllPortsSameDT=off  OutDataTypeStr=boolean
  OR2 : Logic  Operator=OR  AllPortsSameDT=off  OutDataTypeStr=boolean
  Product{,1..5} (6 alike) : Product
  Rate Limiter Dynamic{,1..6} (7 alike) : simulink/Discontinuities/Rate Limiter Dynamic
      settings: SourceProductName=Simulink
  Relational Operator : RelationalOperator  Operator=<  OutDataTypeStr=boolean  RndMeth=Simplest
  Relational Operator1 : RelationalOperator  Operator=<  OutDataTypeStr=boolean  RndMeth=Simplest
  Relational Operator9 : RelationalOperator  OutDataTypeStr=boolean  RndMeth=Simplest
  Reset : Constant  Value=single(0)
  ResetDelay : Constant  Value=single(1)
  Saturation : Saturate  UpperLimit=5000  LowerLimit=-5000
  Saturation Dynamic{,1..7} (8 alike) : simulink/Discontinuities/Saturation Dynamic  OutMin=[]  OutMax=[]  OutDataTypeStr=Inherit: Same as second input  OutDataType=fixdt(1, 16)  OutScaling=2^-10  DoSatur=off
  Saturation1 : Saturate  UpperLimit=100  LowerLimit=0
  Saturation2 : Saturate  UpperLimit=100  LowerLimit=0
  Saturation3 : Saturate  UpperLimit=0.7  LowerLimit=0.1
  Steptime : Constant  Value=single(0.01)
  Switch{,1..8} (9 alike) : Switch  Criteria=u2 ~= 0
  Terminator : Terminator
  Terminator1 : Terminator
  Unit Delay{,1..6} (7 alike) : UnitDelay  SampleTime=-1  HasFrameUpgradeWarning=on
  Wtarget : MATLAB Function  TreatAsAtomicUnit=on
  载荷转移 : MATLAB Function  TreatAsAtomicUnit=on
  TrqFL_Final : Outport
  TrqFR_Final : Outport  Port=2
  TrqR_Final : Outport  Port=3
  TVD_Tigger : Outport  Port=4
  wires:
  Gain6/1 -> Rate Limiter Dynamic/3
  [additional_TrqFR] -> Add5/2  "additional_TrqFR"
  Product2/1 -> [FrontTrqRequest_raw]
  Constant34/1 -> Rate Limiter Dynamic4/1, Gain7/1
  AND/1 -> Logical Operator4/2  "DYC_Tigger"
  Add17/1 -> Product1/2
  Gain/1 -> Min1/1, [FLTrqLimit], Saturation Dynamic/1  "FLTrqLimit"
  Constant42/1 -> Add12/3
  Constant43/1 -> Add11/3
  Gain27/1 -> Saturation Dynamic6/3
  Saturation Dynamic1/1 -> Add12/1
  Gain26/1 -> Saturation Dynamic6/1, Gain27/1, Gain28/1, Saturation Dynamic7/1
  Gain9/1 -> Cos1/1
  TrqRequest/1 -> Product2/1, Product1/1
  Saturation Dynamic6/1 -> [additional_TrqFL]  "Frnt_Rear_Adjust_R"
  [FF_Mz] -> Add1/3
  [ax_mpss] -> Gain21/1
  Vx_mps/1 -> Wtarget/1(Vx_mps), [Vx_mps]  "Vx_mps"
  Gain24/1 -> Saturation Dynamic7/2
  [DYC_Actv] -> OR2/1
  Wtarget/1(Wtarget) -> Rate Limiter Dynamic4/2  "Wtarget"
  Gain25/1 -> Saturation Dynamic6/2
  Gain22/1 -> Rate Limiter Dynamic6/3
  Gain21/1 -> Wtarget/9(Ax_mpss)
  Constant45/1 -> Gain23/1, Rate Limiter Dynamic5/1
  Switch1/1 -> Product4/1, Product3/2
  Abs2/1 -> Compare To Constant4/1
  Logical Operator4/1 -> Logical Operator5/1
  Rate Limiter Dynamic5/1 -> [Frnt_Rear_Adjust_F]  "Frnt_Rear_Adjust_F"
  Unit Delay1/1 -> Product5/1
  Constant16/1 -> Wtarget/5(m)
  Gain20/1 -> Saturation2/1
  WSAV/1 -> 2-D Lookup Table/2, MATLAB Function1/2(WSAV)
  Rate Limiter Dynamic1/1 -> TrqFR_Final/1  "TrqFR_Final"
  Min/1 -> Unit Delay4/1, Relational Operator9/1
  228/1 -> MATLAB Function/7(Temrax_max)  "EmraxMaxTroque"
  [Frnt_Rear_Adjust_R] -> Add12/2, Add11/2
  [Front_flag] -> NOT/1
  Relational Operator9/1 -> Logical Operator5/2
  Add18/1 -> Saturation3/1
  [WhlStrAng] -> Abs5/1
  WhlStrAng/1 -> Product/1, Unit Delay2/1, Abs4/1, [WhlStrAng], Wtarget/2(WhlStrAng), MATLAB Function1/1(WSA)
  Saturation3/1 -> Gain4/1, Add17/2  "Frnt_Rear_Adjust_F"
  Saturation1/1 -> Rate Limiter Dynamic5/2  "Frnt_Rear_Adjust_F"
  [Front_flag] -> AND2/1
  Cos3/1 -> Gain12/1
  Gain17/1 -> Rate Limiter Dynamic2/3
  [FRTrqLimit] -> Saturation Dynamic4/1
  Compare To Constant4/1 -> OR/1
  Constant47/1 -> Add17/1
  OR/1 -> Switch6/2
  MATLAB Function/1(T1max) -> Gain/1
  Saturation Dynamic4/1 -> Rate Limiter Dynamic1/2  "TrqFR_Final"
  Gain28/1 -> Saturation Dynamic7/3
  [Vx_mps] -> 2-D Lookup Table1/2
  Gain5/1 -> Rate Limiter Dynamic3/3
  Constant48/1 -> Gain5/1, Rate Limiter Dynamic3/1
  Divide1/1 -> Gain25/1
  Rate Limiter Dynamic/1 -> TrqFL_Final/1  "TrqFL_Final"
  [FrontTrqRequest_raw] -> Gain26/1
  Constant3/1 -> 载荷转移/4(lfw)
  MATLAB Function/2(T2max) -> Gain1/1
  [FRTrqLimit] -> Min1/2
  NOT1/1 -> Switch5/2
  Product/1 -> Compare To Constant/1
  Gain13/1 -> Add9/1
  Logical Operator3/1 -> Switch3/2
  MATLAB Function/3(T34max) -> Gain2/1
  [Vx_mps] -> MATLAB Function1/3(Vx)
  [Rear_flag] -> AND1/2
  Unit Delay2/1 -> Product/2
  Relational Operator1/1 -> [Rear_flag]  "Rear_flag"
  [RTrqLimit] -> Divide3/2
  Constant12/1 -> MATLAB Function/10(i1)
  Constant35/1 -> Product4/2
  Constant40/1 -> Switch8/3
  Unit Delay3/1 -> Logical Operator4/1
  Wactul/1 -> Add/1, [Wactul]  "Wactul"
  Constant4/1 -> 载荷转移/5(lrw)
  Constant23/1 -> MATLAB Function1/7(lf)
  Constant8/1 -> Saturation Dynamic2/3
  [Vx_mps] -> Compare To Constant3/1
  AND3/1 -> Switch1/2
  Min1/1 -> Divide3/1, Add14/1
  [Front_flag] -> AND1/1
  Add12/1 -> Saturation Dynamic4/2
  [Mz_Raw] -> Divide2/1
  Gain11/1 -> Add7/1
  Gain10/1 -> Add7/2
  Switch5/1 -> Switch2/3
  Constant44/1 -> Gain22/1, Rate Limiter Dynamic6/1
  Constant24/1 -> MATLAB Function1/8(lr)
  ay_mpss/1 -> 载荷转移/2(ay), [ay_mpss]  "ay_mpss"
  Add1/1 -> Saturation/1, Add3/2
  [Rear_flag] -> AND2/2
  载荷转移/1(Fz1) -> MATLAB Function/1(Fz1)  "Fz1"
  FRWhlStrAng/1 -> Gain14/1, Add8/1
  Cos2/1 -> Gain13/1
  AND2/1 -> OR2/2
  Wtarget/2(btarget) -> Terminator/1
  Gain16/1 -> Rate Limiter Dynamic1/3
  FLWhlStrAng/1 -> Add6/1, Gain8/1
  Constant22/1 -> MATLAB Function1/4(Iz)
  Compare To Constant/1 -> [cross_zore]
  [Mz_Raw] -> Divide1/1
  MATLAB Function1/1(Mz) -> Switch4/1
  Add14/1 -> Relational Operator/1, Switch5/1
  [RearTrqRequest_raw] -> Saturation Dynamic2/2, Add15/2
  Gain12/1 -> Add9/2
  Reset/1 -> Switch6/3
  Relational Operator/1 -> [Front_flag]  "Front_flag"
  Saturation Dynamic3/1 -> Rate Limiter Dynamic/2  "TrqFL_Final"
  Add/1 -> [Werror], Switch1/1  "Werror"
  Compare To Constant3/1 -> AND/3
  Add3/1 -> Unit Delay1/1
  AND1/1 -> OR1/2
  Unit Delay4/1 -> Add10/1
  Constant17/1 -> Wtarget/6(Car)
  Divide3/1 -> Add18/1  "k"
  Constant31/1 -> Saturation Dynamic5/3
  Add9/1 -> Divide2/2
  Logical Operator5/1 -> TVD_Tigger/1, [DYC_Actv], Unit Delay3/1  "DYC_Actv"
  Constant29/1 -> Saturation Dynamic3/3
  Constant7/1 -> Saturation Dynamic1/3
  Product5/1 -> Add2/3
  [DYC_Actv] -> OR1/1
  Constant2/1 -> 载荷转移/3(h)
  Gain23/1 -> Rate Limiter Dynamic5/3
  Unit Delay5/1 -> Switch3/3
  Constant/1 -> Switch/1
  [ax_mpss] -> Compare To Constant5/1
  Saturation Dynamic2/1 -> Add13/1
  Compare To Constant1/1 -> AND/1
  Add7/1 -> Divide1/2
  amkFL_rpm/1 -> AMK/1
  Add15/1 -> Switch8/1, Relational Operator1/1
  Constant26/1 -> MATLAB Function/12(u)
  Rate Limiter Dynamic2/1 -> TrqR_Final/1  "TrqR_Final"
  Switch/1 -> Add2/1
  Abs4/1 -> 2-D Lookup Table/1
  Divide2/1 -> Gain24/1
  Constant1/1 -> Switch1/3
  Constant6/1 -> Saturation Dynamic/3
  Gain8/1 -> Cos/1
  Constant21/1 -> MATLAB Function1/5(Caf)
  [DYC_Actv] -> Unit Delay6/1, Switch4/2
  Compare To Constant5/1 -> OR/2
  Constant27/1 -> Add6/2
  Add5/1 -> Saturation Dynamic1/2
  OR1/1 -> Switch2/2
  Constant33/1 -> Switch5/3
  Switch7/1 -> Gain20/1
  载荷转移/3(Fz3) -> MATLAB Function/3(Fz3)  "Fz3"
  Constant30/1 -> Saturation Dynamic4/3
  Cos1/1 -> Gain10/1
  Abs/1 -> Compare To Constant1/1
  [Werror] -> Abs/1
  Add10/1 -> Switch6/1
  Constant39/1 -> Switch7/1
  Gain2/1 -> [RTrqLimit], Add15/1, Saturation Dynamic5/1, Saturation Dynamic2/1  "RTrqLimit"
  Product1/1 -> [RearTrqRequest_raw]
  [Wactul] -> Abs1/1
  Constant5/1 -> 载荷转移/6(lf)
  Unit Delay6/1 -> Logical Operator3/1
  Add8/1 -> Gain15/1
  Add4/1 -> Add14/2, Saturation Dynamic/2
  Steptime/1 -> Add10/2
  Constant14/1 -> Wtarget/3(lf)
  Gain14/1 -> Cos2/1
  Gain15/1 -> Cos3/1
  Compare To Constant2/1 -> AND/2
  [Frnt_Rear_Adjust_F] -> Add13/2  "Frnt_Rear_Adjust_F"
  Constant41/1 -> Rate Limiter Dynamic/1, Gain6/1, Rate Limiter Dynamic1/1, Gain16/1, Gain17/1, Rate Limiter Dynamic2/1
  Gain19/1 -> Saturation1/1
  Add6/1 -> Gain9/1
  Constant32/1 -> Switch2/1
  Constant36/1 -> Product5/2
  AMK/1 -> MATLAB Function/5(TamkFL_max)  "AMKMaxTroqueFL"
  AMK1/1 -> MATLAB Function/6(TamkFR_max)  "AMKMaxTroqueFL"
  载荷转移/4(Fz4) -> MATLAB Function/4(Fz4)  "Fz4"
  Constant11/1 -> MATLAB Function/9(Rt)
  ax_mpss/1 -> [ax_mpss], 载荷转移/1(ax)  "ax_mpss"
  Constant18/1 -> Wtarget/7(Caf)
  Saturation Dynamic5/1 -> Rate Limiter Dynamic2/2  "TrqR_Final"
  Constant9/1 -> 载荷转移/7(lr)
  Switch4/1 -> Switch3/1
  Constant37/1 -> Relational Operator/2
  Saturation Dynamic7/1 -> [additional_TrqFR]  "Frnt_Rear_Adjust_R"
  Add2/1 -> Add1/2, Unit Delay/1
  emrax_rpm/1 -> 228/1
  Constant13/1 -> MATLAB Function/11(i2)
  Constant46/1 -> Product3/1  "Kp"
  ResetDelay/1 -> Relational Operator9/2, Min/2
  [FrontTrqRequest_raw] -> Add5/1, Add4/1
  amkFR_rpm/1 -> AMK1/1
  Cos/1 -> Gain11/1
  Constant15/1 -> Wtarget/4(lr)
  Rate Limiter Dynamic4/1 -> Add/2  "Wtarget"
  [additional_TrqFL] -> Add4/2  "additional_TrqFL"
  Saturation/1 -> [Mz_Raw], Add3/1  "Mz_Raw"
  Saturation2/1 -> Rate Limiter Dynamic6/2  "Frnt_Rear_Adjust_R"
  [FLTrqLimit] -> Saturation Dynamic3/1
  Abs1/1 -> Compare To Constant2/1
  Constant28/1 -> Add8/2
  Add11/1 -> Saturation Dynamic3/2
  InitZORE/1 -> Switch4/3
  Gain7/1 -> Rate Limiter Dynamic4/3
  [cross_zore] -> Switch/2
  Product3/1 -> Add1/1
  NOT/1 -> Switch8/2
  Unit Delay/1 -> Switch/3
  Abs5/1 -> 2-D Lookup Table1/1
  2-D Lookup Table1/1 -> Rate Limiter Dynamic3/2  "K"
  Switch2/1 -> Gain19/1
  Product4/1 -> Add2/2
  载荷转移/2(Fz2) -> MATLAB Function/2(Fz2)  "Fz2"
  Switch6/1 -> Min/1
  Switch3/1 -> [FF_Mz], Unit Delay5/1  "FF_Mz"
  Constant20/1 -> MATLAB Function1/6(Car)
  Gain4/1 -> Product2/2
  [Rear_flag] -> NOT1/1
  Rate Limiter Dynamic6/1 -> [Frnt_Rear_Adjust_R]  "Frnt_Rear_Adjust_R"
  Constant25/1 -> MATLAB Function1/9(m)
  Constant38/1 -> Relational Operator1/2
  Constant19/1 -> Wtarget/8(u)
  [ay_mpss] -> Gain3/1
  Gain3/1 -> MATLAB Function/8(ay_g)
  Gain1/1 -> [FRTrqLimit], Saturation Dynamic1/1  "FRTrqLimit"
  OR2/1 -> Switch7/2
  Saturation Dynamic/1 -> Add11/1
  Switch8/1 -> Switch7/3
  Rate Limiter Dynamic3/1 -> Add18/2  "K"
  Add13/1 -> Saturation Dynamic5/2
  Constant10/1 -> 载荷转移/8(m)
  2-D Lookup Table/1 -> Terminator1/1
  [Werror] -> Abs2/1
  [DYC_Actv] -> AND3/2
  DYC_Enable/1 -> AND3/1
